simulink model "sampleModel1870"  (R2023a)
settings: Solver=VariableStepAuto  StartTime=0.0  StopTime=10.0  RelTol=1e-3
libraries: hdlsllib x5, simulink x3
settings Model: Creator=user1  LastModifiedBy=user1

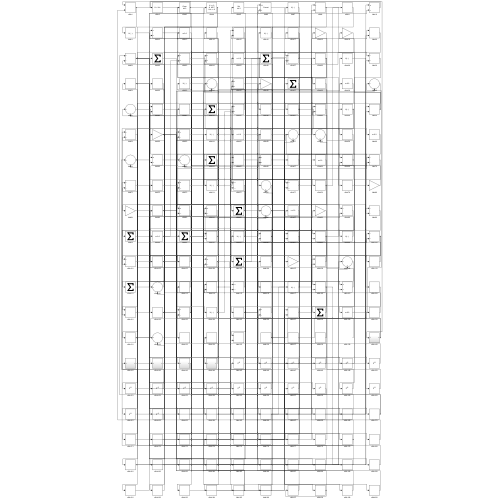
[thumbnail: Simulink's stored preview of the top-level diagram]
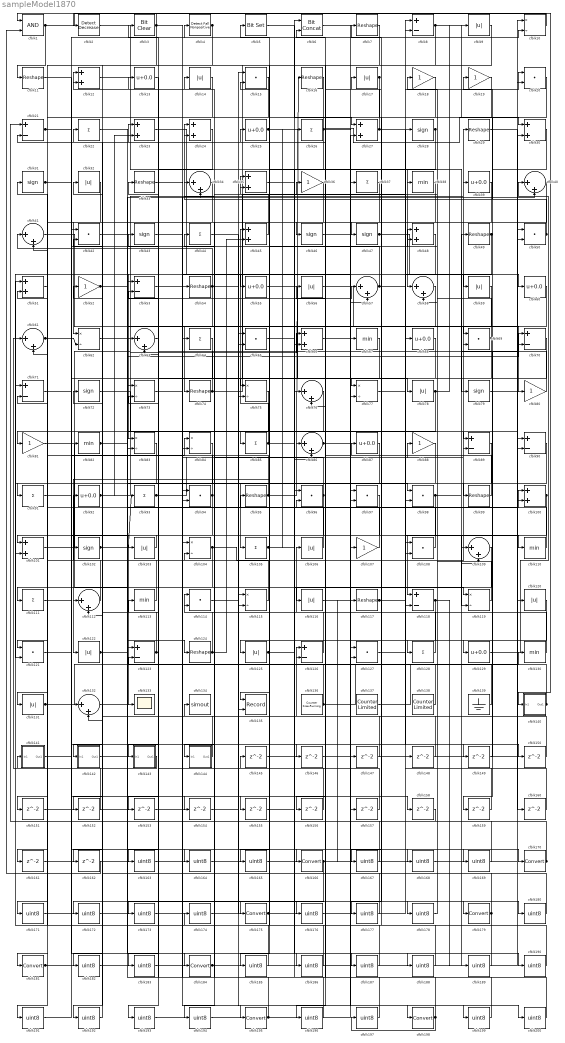
== system sampleModel1870 ==
  cfblk1 : Logic  AllPortsSameDT=off  OutDataTypeStr=boolean
  cfblk{10,62,73,75,77,83..84,104,115,119} (10 alike) : Product  Inputs=*/  RndMeth=Zero  SaturateOnIntegerOverflow=on
  cfblk{12,23..24,27,30,35,45,48,51,66,100..101} (12 alike) : Sum
  cfblk{28,31,43,46..47,72,79,102} (8 alike) : Signum
  cfblk{9,14,17,32,56,59,78,103,106,116,120,122,125,131} (14 alike) : Abs  SaturateOnIntegerOverflow=off
  cfblk{22,26,37,44,64,85,91,93,105,111,128} (11 alike) : Sum  Inputs=+
  cfblk{18..19,36,52,80..81,88,107} (8 alike) : Gain
  cfblk{15,20,42,50,65,69,94,96..98,108,114,121,127} (14 alike) : DotProduct  OutDataTypeStr=Inherit: Inherit via internal rule
  cfblk{34,40..41,57..58,61,63,76,86,109,112,132} (12 alike) : Sum  Inputs=|++
  cfblk{7,11,16,29,33,49,54,74,95,99,117,124} (12 alike) : Reshape
  cfblk{38,67,82,110,113,130} (6 alike) : MinMax
  cfblk{8,21,53,70..71,89..90,118,123,126} (10 alike) : Sum  Inputs=+-
  cfblk{13,25,39,55,60,68,87,92,129} (9 alike) : Bias  Bias=0.0  SaturateOnIntegerOverflow=off
  cfblk133 : Scope
  cfblk134 : ToWorkspace  VariableName=simout  SaveFormat=Timeseries  SampleTime=-1
  cfblk135 : Record  FileSettingsInternal="{\"entries\":[{\"content\":{\"excelSettings\":{\"content\":{},\"type\":\"Streamout.ExcelSettings\"}},\"type\":\"Streamout.FileSettingStorage\",\"uuid\":\"\"}],\"packageUris\":[\"http:\\/\\/schema.mathworks.com\\/mf0\\/streamout_blocks\\/R2020a\"],\"version\":\"1.0\"}"  Layout=[1 1]  SignalsInternal="{\"entries\":[{\"content\":{\"signals\":[{\"content\":{\"blockPath\":[],\"dimensions\":[1],\"domain\":\"\",\"lineColor\":\"#a2142f\",\"plots\":[1],\"port\":1,\"signalID\":4646,\"signalName\":\"XY Graph:1\"},\"type\":\"RecordBlkView.Signal\",\"uuid\":\"\"},{\"content\":{\"blockPath\":[],\"dimensions\":[1],\"domain\":\"\",\"lineColor\":\"#139fff\",\"plots\":[1],\"port\":2,\"signalID\":4649,\"signalName\":\"XY Graph:2\"},\"type\":\"RecordBlkView.Signal\",\"uuid\":\"\"}]},\"type\":\"RecordBlkView.InputSignals\",\"uuid\":\"\"}],\"packageUris\":[\"http:\\/\\/schema.mathworks.com\\/mf0\\/streamout_blocks\\/R2020a\"],\"version\":\"1.0\"}"  VisualizationBindings="{\"xyplotplugin\":{\"info\":[{\"series\":[{\"bindingParametersList\":[{\"parameter\":\"X-Axis\",\"signalID\":4646,\"signalName\":\"XY Graph:1\"},{\"parameter\":\"Y-Axis\",\"signalID\":4649,\"signalName\":\"XY Graph:2\"}],\"seriesID\":29567}],\"subplotID\":1}]}}"  CompatibilityTag=XY  st=-1
  cfblk136 : hdlsllib/Sources/Counter Free-Running  NumBits=16  tsamp=-1
  cfblk137 : hdlsllib/Sources/Counter Limited  uplimit=7  tsamp=-1
  cfblk138 : hdlsllib/Sources/Counter Limited  uplimit=7  tsamp=-1
  cfblk139 : Ground
  cfblk140 : Subsystem
      settings: LibrarySourceBlock=|
      | hdlsllib/Ports &
      | Subsystems/Subsystem
  cfblk141 : Subsystem
      settings: LibrarySourceBlock=|
      | hdlsllib/Ports &
      | Subsystems/Subsystem
  cfblk142 : Subsystem
      settings: LibrarySourceBlock=|
      | hdlsllib/Ports &
      | Subsystems/Subsystem
  cfblk143 : Subsystem
      settings: LibrarySourceBlock=|
      | hdlsllib/Ports &
      | Subsystems/Subsystem
  cfblk144 : Subsystem
      settings: LibrarySourceBlock=|
      | hdlsllib/Ports &
      | Subsystems/Subsystem
  cfblk{145..162} (18 alike) : Delay  SampleTime=1
  cfblk{163..165,167..169,171..174,176..178,180,182..183,185..194,196..197,199..200} (30 alike) : DataTypeConversion  OutDataTypeStr=uint8  SaturateOnIntegerOverflow=off  RndMeth=Floor
  cfblk{166,170,175,179,181,184,195,198} (8 alike) : DataTypeConversion  SaturateOnIntegerOverflow=off  RndMeth=Floor
  cfblk2 : simulink/Logic and Bit Operations/Detect Decrease  vinit=0.0  OutDataTypeStr=boolean
      settings: LibrarySourceBlock=|
      | hdlsllib/Logic and Bit
      | Operations/Detect
      | Decrease
  cfblk3 : simulink/Logic and Bit Operations/Bit Clear  iBit=0
      settings: LibrarySourceBlock=|
      | hdlsllib/Logic and Bit
      | Operations/Bit Clear
  cfblk4 : hdlsllib/Logic and Bit Operations/Detect Fall Nonpositive  vinit=0  OutDataTypeStr=boolean
  cfblk5 : simulink/Logic and Bit Operations/Bit Set  iBit=0
      settings: LibrarySourceBlock=|
      | hdlsllib/Logic and Bit
      | Operations/Bit Set
  cfblk6 : hdlsllib/Logic and Bit Operations/Bit Concat  numInputs=2
  wires:
  cfblk88/1 -> cfblk105/1
  cfblk55/1 -> cfblk78/1
  cfblk95/1 -> cfblk16/1, cfblk31/1
  cfblk85/1 -> cfblk45/1, cfblk188/1
  cfblk104/1 -> cfblk29/1, cfblk161/1
  cfblk27/1 -> cfblk122/1, cfblk110/1
  cfblk98/1 -> cfblk133/1, cfblk70/1
  cfblk32/1 -> cfblk62/1
  cfblk14/1 -> cfblk143/1(In1)
  cfblk16/1 -> cfblk129/1
  cfblk92/1 -> cfblk66/1, cfblk23/2
  cfblk108/1 -> cfblk56/1
  cfblk7/1 -> cfblk112/1
  cfblk41/1 -> cfblk80/1
  cfblk65/1 -> cfblk170/1
  cfblk113/1 -> cfblk32/1
  cfblk110/1 -> cfblk36/1
  cfblk123/1 -> cfblk52/1, cfblk23/1
  cfblk72/1 -> cfblk89/1
  cfblk58/1 -> cfblk74/1
  cfblk34/1 -> cfblk111/1
  cfblk54/1 -> cfblk41/1, cfblk90/2, cfblk183/1
  cfblk101/1 -> cfblk39/1
  cfblk126/1 -> cfblk106/1
  cfblk100/1 -> cfblk118/1, cfblk119/2
  cfblk129/1 -> cfblk40/1
  cfblk73/1 -> cfblk54/1
  cfblk139/1 -> cfblk17/1
  cfblk87/1 -> cfblk125/1
  cfblk1/1 -> cfblk140/1(In1), cfblk11/1
  cfblk8/1 -> cfblk135/1, cfblk30/1
  cfblk103/1 -> cfblk101/1
  cfblk142/1(Out1) -> cfblk40/2
  cfblk130/1 -> cfblk35/1
  cfblk23/1 -> cfblk107/1
  cfblk38/1 -> cfblk116/1
  cfblk67/1 -> cfblk175/1
  cfblk12/1 -> cfblk76/1
  cfblk48/1 -> cfblk83/1
  cfblk39/1 -> cfblk47/1
  cfblk144/1(Out1) -> cfblk134/1
  cfblk137/1 -> cfblk49/1
  cfblk20/1 -> cfblk142/1(In1)
  cfblk42/1 -> cfblk184/1
  cfblk81/1 -> cfblk123/1
  cfblk28/1 -> cfblk156/1, cfblk165/1
  cfblk61/1 -> cfblk62/2, cfblk151/1
  cfblk143/1(Out1) -> cfblk61/1
  cfblk30/1 -> cfblk99/1
  cfblk13/1 -> cfblk63/1
  cfblk112/1 -> cfblk92/1
  cfblk6/1 -> cfblk198/1
  cfblk24/1 -> cfblk63/2
  cfblk21/1 -> cfblk103/1, cfblk4/1, cfblk146/1, cfblk186/1
  cfblk93/1 -> cfblk89/2, cfblk88/1
  cfblk102/1 -> cfblk93/1, cfblk70/2
  cfblk52/1 -> cfblk84/2, cfblk124/1, cfblk162/1, cfblk180/1
  cfblk2/1 -> cfblk58/1
  cfblk118/1 -> cfblk185/1, cfblk189/1
  cfblk131/1 -> cfblk130/1, cfblk48/2
  cfblk10/1 -> cfblk2/1
  cfblk136/1 -> cfblk5/1, cfblk50/2, cfblk57/2
  cfblk80/1 -> cfblk12/1
  cfblk51/1 -> cfblk81/1
  cfblk84/1 -> cfblk101/2
  cfblk125/1 -> cfblk96/1, cfblk100/2
  cfblk47/1 -> cfblk59/1, cfblk167/1
  cfblk111/1 -> cfblk10/2
  cfblk122/1 -> cfblk100/1, cfblk154/1
  cfblk9/1 -> cfblk46/1
  cfblk50/1 -> cfblk24/1, cfblk19/1
  cfblk105/1 -> cfblk118/2, cfblk26/1
  cfblk53/1 -> cfblk195/1
  cfblk22/1 -> cfblk179/1
  cfblk31/1 -> cfblk77/2, cfblk158/1
  cfblk127/1 -> cfblk28/1
  cfblk117/1 -> cfblk20/1, cfblk7/1
  cfblk128/1 -> cfblk24/2
  cfblk107/1 -> cfblk44/1
  cfblk69/1 -> cfblk35/2, cfblk75/1
  cfblk116/1 -> cfblk97/1
  cfblk97/1 -> cfblk102/1
  cfblk138/1 -> cfblk3/1
  cfblk36/1 -> cfblk144/1(In1)
  cfblk5/1 -> cfblk27/1
  cfblk78/1 -> cfblk91/1, cfblk9/1
  cfblk109/1 -> cfblk181/1
  cfblk86/1 -> cfblk27/2, cfblk98/2
  cfblk120/1 -> cfblk128/1
  cfblk124/1 -> cfblk114/1, cfblk45/2
  cfblk76/1 -> cfblk83/2
  cfblk94/1 -> cfblk131/1, cfblk72/1
  cfblk106/1 -> cfblk51/2
  cfblk115/1 -> cfblk41/2
  cfblk56/1 -> cfblk69/1
  cfblk64/1 -> cfblk94/2
  cfblk90/1 -> cfblk135/2
  cfblk99/1 -> cfblk21/2
  cfblk3/1 -> cfblk1/1, cfblk55/1, cfblk192/1
  cfblk25/1 -> cfblk79/1, cfblk38/1
  cfblk26/1 -> cfblk85/1, cfblk119/1
  cfblk79/1 -> cfblk120/1
  cfblk40/1 -> cfblk77/1
  cfblk74/1 -> cfblk8/2, cfblk13/1
  cfblk63/1 -> cfblk43/1
  cfblk4/1 -> cfblk171/1, cfblk182/1
  cfblk91/1 -> cfblk84/1
  cfblk96/1 -> cfblk34/1, cfblk115/2
  cfblk121/1 -> cfblk82/1
  cfblk17/1 -> cfblk97/2, cfblk86/1
  cfblk140/1(Out1) -> cfblk126/1, cfblk104/2
  cfblk45/1 -> cfblk12/2
  cfblk119/1 -> cfblk48/1
  cfblk44/1 -> cfblk115/1
  cfblk82/1 -> cfblk57/1, cfblk98/1
  cfblk57/1 -> cfblk60/1, cfblk25/1
  cfblk19/1 -> cfblk61/2
  cfblk49/1 -> cfblk121/1, cfblk121/2
  cfblk141/1(Out1) -> cfblk166/1
  cfblk145/1 -> cfblk108/2
  cfblk146/1 -> cfblk10/1
  cfblk147/1 -> cfblk96/2
  cfblk148/1 -> cfblk126/2
  cfblk77/1 -> cfblk149/1
  cfblk149/1 -> cfblk69/2
  cfblk62/1 -> cfblk150/1
  cfblk150/1 -> cfblk112/2
  cfblk151/1 -> cfblk75/2
  cfblk83/1 -> cfblk152/1
  cfblk152/1 -> cfblk51/1
  cfblk89/1 -> cfblk153/1
  cfblk153/1 -> cfblk34/2
  cfblk43/1 -> cfblk155/1
  cfblk155/1 -> cfblk66/2
  cfblk156/1 -> cfblk73/2
  cfblk157/1 -> cfblk123/2
  cfblk158/1 -> cfblk21/1
  cfblk70/1 -> cfblk159/1
  cfblk159/1 -> cfblk58/2
  cfblk29/1 -> cfblk160/1
  cfblk160/1 -> cfblk8/1
  cfblk161/1 -> cfblk30/2
  cfblk162/1 -> cfblk1/2
  cfblk15/1 -> cfblk163/1
  cfblk163/1 -> cfblk64/1
  cfblk11/1 -> cfblk164/1
  cfblk164/1 -> cfblk15/1
  cfblk165/1 -> cfblk15/2
  cfblk166/1 -> cfblk148/1, cfblk117/1, cfblk172/1
  cfblk167/1 -> cfblk141/1(In1)
  cfblk33/1 -> cfblk168/1
  cfblk168/1 -> cfblk20/2
  cfblk46/1 -> cfblk169/1
  cfblk169/1 -> cfblk33/1
  cfblk170/1 -> cfblk76/2, cfblk113/1
  cfblk171/1 -> cfblk65/1
  cfblk172/1 -> cfblk65/2
  cfblk68/1 -> cfblk173/1
  cfblk173/1 -> cfblk127/2
  cfblk174/1 -> cfblk68/1
  cfblk175/1 -> cfblk157/1, cfblk127/1
  cfblk114/1 -> cfblk176/1
  cfblk176/1 -> cfblk67/1
  cfblk18/1 -> cfblk177/1
  cfblk177/1 -> cfblk145/1
  cfblk35/1 -> cfblk178/1
  cfblk178/1 -> cfblk18/1
  cfblk179/1 -> cfblk174/1, cfblk108/1
  cfblk180/1 -> cfblk22/1
  cfblk181/1 -> cfblk86/2, cfblk94/1
  cfblk182/1 -> cfblk109/1
  cfblk183/1 -> cfblk109/2
  cfblk184/1 -> cfblk114/2, cfblk90/1, cfblk50/1
  cfblk185/1 -> cfblk42/1
  cfblk186/1 -> cfblk42/2
  cfblk71/1 -> cfblk187/1
  cfblk187/1 -> cfblk95/1
  cfblk188/1 -> cfblk71/1
  cfblk189/1 -> cfblk71/2
  cfblk132/1 -> cfblk190/1
  cfblk190/1 -> cfblk87/1
  cfblk75/1 -> cfblk191/1
  cfblk191/1 -> cfblk132/1
  cfblk192/1 -> cfblk132/2
  cfblk37/1 -> cfblk193/1
  cfblk193/1 -> cfblk147/1
  cfblk59/1 -> cfblk194/1
  cfblk194/1 -> cfblk37/1
  cfblk195/1 -> cfblk104/1, cfblk73/1
  cfblk60/1 -> cfblk196/1
  cfblk196/1 -> cfblk53/1
  cfblk197/1 -> cfblk53/2
  cfblk198/1 -> cfblk197/1, cfblk14/1
  cfblk66/1 -> cfblk199/1
  cfblk199/1 -> cfblk6/1
  cfblk154/1 -> cfblk200/1
  cfblk200/1 -> cfblk6/2

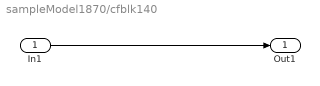
== system sampleModel1870/cfblk140 ==
  In1 : Inport
  Out1 : Outport
  wires:
  In1/1 -> Out1/1

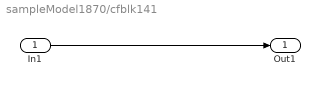
== system sampleModel1870/cfblk141 ==
  In1 : Inport
  Out1 : Outport
  wires:
  In1/1 -> Out1/1

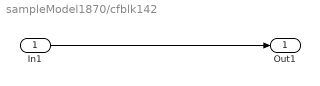
== system sampleModel1870/cfblk142 ==
  In1 : Inport
  Out1 : Outport
  wires:
  In1/1 -> Out1/1

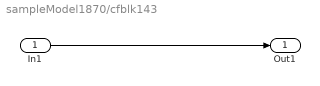
== system sampleModel1870/cfblk143 ==
  In1 : Inport
  Out1 : Outport
  wires:
  In1/1 -> Out1/1

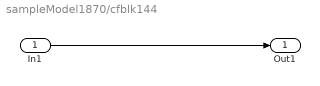
== system sampleModel1870/cfblk144 ==
  In1 : Inport
  Out1 : Outport
  wires:
  In1/1 -> Out1/1
